simulink model "SMA_model"  (R2021b)
settings: Solver=VariableStepAuto  StartTime=0.0  StopTime=10.0  RelTol=1e-3
values from neighbouring files (symbols this model uses):
  A_f = 98    [init.m]
  A_s = 88    [init.m]
  A_w = 290.45e-6    (= 0.00029045)    [init.m]
  C_A = 10e6    (= 10000000)    [init.m]
  C_M = 10e6    (= 10000000)    [init.m]
  c_p = 320    [init.m]
  E_A = 75e9    (= 75000000000)    [init.m]
  E_M = 28e9    (= 28000000000)    [init.m]
  epsilon_L = 0.023    [init.m]
  h_0 = 20    [init.m]
  h_2 = 0.001    [init.m]
  M_f = 62    [init.m]
  M_s = 72    [init.m]
  m_w = 6.8e-4    (= 0.00068)    [init.m]
  R = 20    [init.m]
  T_amb = 25    [init.m]
  Theta = -0.055    [init.m]
settings Model: Creator=Raj Shah  LastModifiedBy=Raj Shah

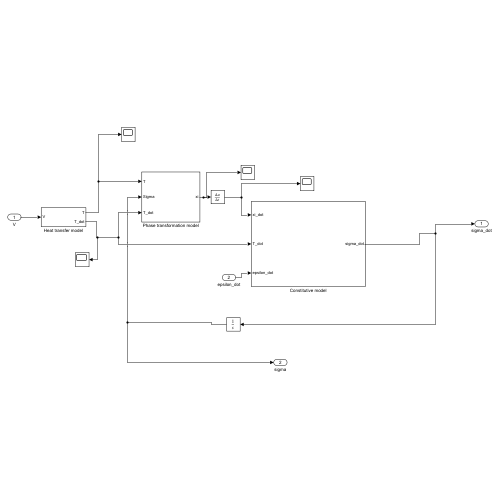
[thumbnail: Simulink's stored preview of the top-level diagram]
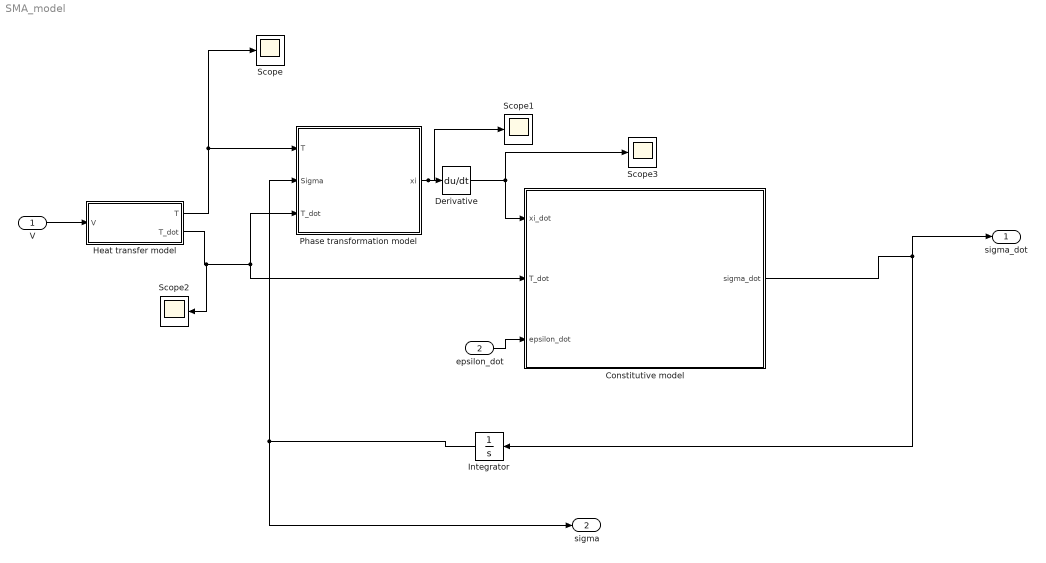
== system SMA_model ==
  V : Inport
  epsilon_dot : Inport  Port=2
  Constitutive model : Subsystem
  Derivative : Derivative
  Heat transfer model : Subsystem
  Integrator : Integrator
  Phase transformation model : Subsystem
  Scope{,1..3} (4 alike) : Scope
  sigma_dot : Outport
  sigma : Outport  Port=2
  wires:
  V/1 -> Heat transfer model/1(V)
  epsilon_dot/1 -> Constitutive model/3(epsilon_dot)
  Heat transfer model/2(T_dot) -> Scope2/1, Phase transformation model/3(T_dot), Constitutive model/2(T_dot)
  Heat transfer model/1(T) -> Scope/1, Phase transformation model/1(T)
  Constitutive model/1(sigma_dot) -> Integrator/1, sigma_dot/1
  Integrator/1 -> sigma/1, Phase transformation model/2(Sigma)
  Phase transformation model/1(xi) -> Scope1/1, Derivative/1
  Derivative/1 -> Scope3/1, Constitutive model/1(xi_dot)

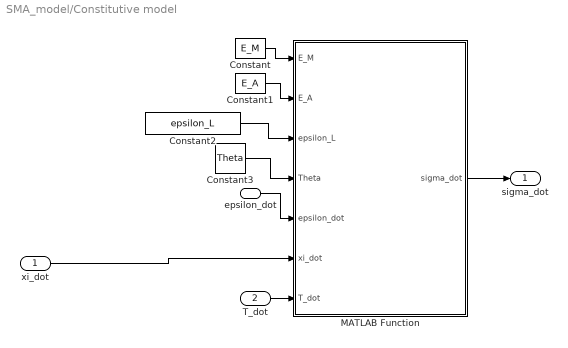
== system SMA_model/Constitutive model ==
  xi_dot : Inport
  T_dot : Inport  Port=2
  epsilon_dot : Inport  Port=3
  Constant : Constant  Value=E_M
  Constant1 : Constant  Value=E_A
  Constant2 : Constant  Value=epsilon_L
  Constant3 : Constant  Value=Theta
  MATLAB Function : MATLAB Function  TreatAsAtomicUnit=on
  sigma_dot : Outport
  wires:
  MATLAB Function/1(sigma_dot) -> sigma_dot/1
  epsilon_dot/1 -> MATLAB Function/5(epsilon_dot)
  xi_dot/1 -> MATLAB Function/6(xi_dot)
  T_dot/1 -> MATLAB Function/7(T_dot)
  Constant/1 -> MATLAB Function/1(E_M)
  Constant1/1 -> MATLAB Function/2(E_A)
  Constant2/1 -> MATLAB Function/3(epsilon_L)
  Constant3/1 -> MATLAB Function/4(Theta)

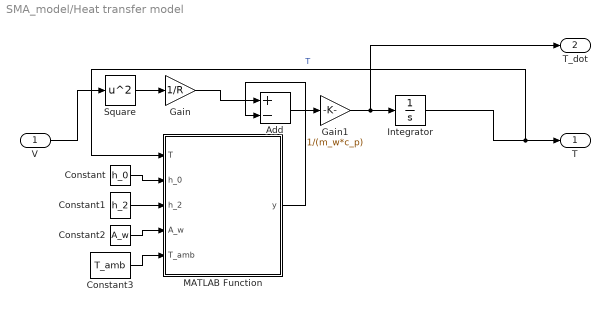
== system SMA_model/Heat transfer model ==
  V : Inport
  Add : Sum  Inputs=+-
  Constant : Constant  Value=h_0
  Constant1 : Constant  Value=h_2
  Constant2 : Constant  Value=A_w
  Constant3 : Constant  Value=T_amb
  Gain : Gain  Gain=1/R
  Gain1 : Gain  Gain=1/(m_w*c_p)
  Integrator : Integrator  InitialCondition=T_amb
  MATLAB Function : MATLAB Function  TreatAsAtomicUnit=on
  Square : Math  Operator=square  SaturateOnIntegerOverflow=on
  T : Outport
  T_dot : Outport  Port=2
  wires:
  V/1 -> Square/1
  Square/1 -> Gain/1
  Gain/1 -> Add/1
  MATLAB Function/1(y) -> Add/2
  Add/1 -> Gain1/1
  Gain1/1 -> T_dot/1, Integrator/1
  Integrator/1 -> MATLAB Function/1(T), T/1  "T"
  Constant/1 -> MATLAB Function/2(h_0)
  Constant1/1 -> MATLAB Function/3(h_2)
  Constant2/1 -> MATLAB Function/4(A_w)
  Constant3/1 -> MATLAB Function/5(T_amb)

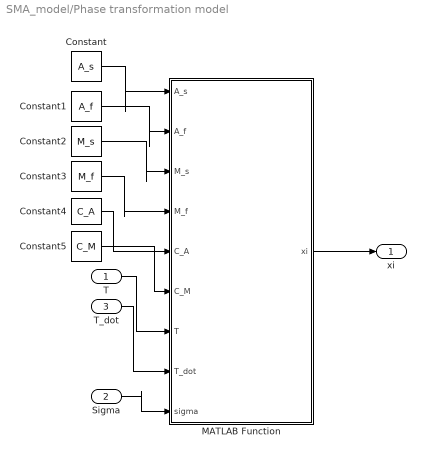
== system SMA_model/Phase transformation model ==
  T : Inport
  Sigma : Inport  Port=2
  T_dot : Inport  Port=3
  Constant : Constant  Value=A_s
  Constant1 : Constant  Value=A_f
  Constant2 : Constant  Value=M_s
  Constant3 : Constant  Value=M_f
  Constant4 : Constant  Value=C_A
  Constant5 : Constant  Value=C_M
  MATLAB Function : MATLAB Function  TreatAsAtomicUnit=on
  xi : Outport
  wires:
  T/1 -> MATLAB Function/7(T)
  Sigma/1 -> MATLAB Function/9(sigma)
  Constant/1 -> MATLAB Function/1(A_s)
  Constant1/1 -> MATLAB Function/2(A_f)
  Constant2/1 -> MATLAB Function/3(M_s)
  Constant3/1 -> MATLAB Function/4(M_f)
  Constant4/1 -> MATLAB Function/5(C_A)
  Constant5/1 -> MATLAB Function/6(C_M)
  T_dot/1 -> MATLAB Function/8(T_dot)
  MATLAB Function/1(xi) -> xi/1

== matlab function SMA_model/Phase transformation model/MATLAB Function ==
  data: A_s input; A_f input; M_s input; M_f input; C_A input; C_M input; T input; T_dot input; xi output; sigma input
function xi = fcn(A_s,A_f,M_s,M_f,C_A,C_M,T,T_dot,sigma)
    A_s_star = A_s + sigma/C_A;
    A_f_star = A_f + sigma/C_A;
    M_s_star = M_s + sigma/C_M;
    M_f_star = M_f + sigma/C_M;
    a_A = pi/(A_f-A_s);
    a_M = pi/(M_s-M_f);
    b_A = -a_A/C_A;
    b_M = -a_M/C_M;

    if(T_dot>=0)
        if(T>A_s_star && T<A_f_star)
%             xi_dot = -1/2*(sin(a_A*(T-A_s)+b_A*sigma))*(a_A*T_dot+b_A*sigma_dot);
            xi = 1/2 * (cos(a_A*(T-A_s)+b_A*sigma)+1);
        elseif(T>=A_s_star)
%             xi_dot = 0;
            xi = 0;
        else
            xi = 1;
        end
    else
         if(T>M_f_star && T<M_s_star)
%              xi_dot = 1/2 * (-sin(a_M*(T-M_f)+b_M*sigma)) * (a_M*T_dot + b_M*sigma_dot);
            xi = 1/2 * (cos(a_M*(T-M_f)+b_M*sigma)+1);
         elseif(T<=M_f_star)
%              xi_dot = 0;
            xi = 1;
         else
            xi = 0;
         end
    end

end

== matlab function SMA_model/Heat transfer model/MATLAB Function ==
  data: T input; y output; h_0 input; h_2 input; A_w input; T_amb input
function y = fcn(T,h_0,h_2,A_w,T_amb)
    h = h_0 + h_2*T*T;
    y = h*A_w*(T-T_amb);
end

== matlab function SMA_model/Constitutive model/MATLAB Function ==
  data: E_M input; E_A input; epsilon_L input; Theta input; epsilon_dot input; sigma_dot output; xi_dot input; T_dot input
function sigma_dot   = fcn(E_M,E_A,epsilon_L,Theta,epsilon_dot,xi_dot,T_dot)
    E = (E_M+E_A)/2;
    Omega = -epsilon_L * E;
    sigma_dot = E*epsilon_dot + Omega*xi_dot + Theta*T_dot;
end
